simulink model "AFE_3L_DCP_DCN"  (R2013b)
settings: Solver=FixedStepDiscrete  SolverMode=SingleTasking  StartTime=0.0  StopTime=0.9  FixedStep=Tpas  RelTol=1e-3
values from neighbouring files (symbols this model uses):
  ASF3 = .5    (= 0.5)    [AFE_FV_Params.m]    (also in AFE_FV_ParamsPV4.m; Params.m)
  Cbus = 330e-3    (= 0.33)    [AFE_FV_Params.m]    (also in AFE_FV_ParamsPV4.m; Params.m)
  DAFE = 0    [AFE_FV_Params.m]    (also in AFE_FV_ParamsPV4.m; Params.m)
  fmod4Q = 1e3    (= 1000)    [AFE_FV_Params.m]    (also in AFE_FV_ParamsPV4.m; Params.m)
  Freq = 50    [AFE_FV_Params.m]    (also in AFE_FV_ParamsPV4.m; Params.m)
  IAFE3L = (PAFE3L+Numd(2)/Dend(1))/Ts    [AFE_FV_Params.m]    (also in AFE_FV_ParamsPV4.m = (PAFE3L+NumdAFE(2)/DendAFE(1))/Ts; CalcPIAndFilters.m; Params.m = (PAFE3L+NumdAFE(2)/DendAFE(1))/Ts)
  IDCP = (PDCP+Numd(2)/Dend(1))/Tpas    [AFE_FV_Params.m]    (also in AFE_FV_ParamsPV4.m = (PDCP+Numd(2)/Dend(1))/Ts; CalcPIAndFilters.m = (PDCP+Numd(2)/Dend(1))/Ts; Params.m = (PDCP+Numd(2)/Dend(1))/Ts)
  Kac = 1/(Vac*sqrt(2/3))    [AFE_FV_Params.m]    (also in AFE_FV_ParamsPV4.m; Params.m)
  KLPDCP = mat2str(KLPDCP)    [CalcPIAndFilters.m]
  L = .1    (= 0.1)    [AFE_FV_Params.m]    (also in AFE_FV_ParamsPV4.m; Params.m)
  Lac = 8.1487e-04    (= 0.00081487)    [AFE_FV_Params.m]    (also in AFE_FV_ParamsPV4.m; Params.m)
  Lcoup = 1e-6    (= 1e-06)    [AFE_FV_Params.m]    (also in AFE_FV_ParamsPV4.m = 1e-05; Params.m = 1e-05)
  NAFE = 100    [AFE_FV_Params.m]    (also in AFE_FV_ParamsPV4.m; Params.m)
  PAFE3L = Numd(1)/Dend(1)    [AFE_FV_Params.m]    (also in AFE_FV_ParamsPV4.m = NumdAFE(1)/DendAFE(1); CalcPIAndFilters.m; Params.m = NumdAFE(1)/DendAFE(1))
  PDCP = Numd(1)/Dend(1)    [AFE_FV_Params.m]    (also in AFE_FV_ParamsPV4.m; CalcPIAndFilters.m; Params.m)
  R = .28    (= 0.28)    [AFE_FV_Params.m]    (also in AFE_FV_ParamsPV4.m; Params.m)
  Sat3 = 800    [AFE_FV_Params.m]
  TLPDCP = mat2str(TLPDCP)    [CalcPIAndFilters.m]
  Tpas = 1e-6    (= 1e-06)    [AFE_FV_Params.m]    (also in AFE_FV_ParamsPV4.m; Params.m = 1e-05)
  Vac = 2000    [AFE_FV_Params.m]    (also in AFE_FV_ParamsPV4.m; Params.m)
  Vdc = 5000    [AFE_FV_Params.m]    (also in AFE_FV_ParamsPV4.m; Params.m)
undefined symbols (not defined in the file or in its folder): D1, Delta, Rac
libraries: powerlib x80, simulink x36, powerlib_meascontrol x26
(part 2 of 2)

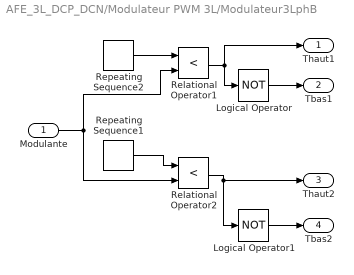
== system AFE_3L_DCP_DCN/Modulateur PWM 3L/Modulateur3LphB ==
  Modulante : Inport
  Logical Operator : Logic  Operator=NOT  AllPortsSameDT=off  OutDataTypeStr=boolean
  Logical Operator1 : Logic  Operator=NOT  AllPortsSameDT=off  OutDataTypeStr=boolean
  Relational Operator1 : RelationalOperator  Operator=<  OutDataTypeStr=boolean
  Relational Operator2 : RelationalOperator  Operator=<  OutDataTypeStr=boolean
  Repeating Sequence1 : simulink/Sources/Repeating Sequence  rep_seq_t=[0 .5/666 1/666]  rep_seq_y=[-1 0 -1]
  Repeating Sequence2 : simulink/Sources/Repeating Sequence  rep_seq_t=[0 .5/666 1/666]  rep_seq_y=[0 1 0]
  Thaut1 : Outport
  Tbas1 : Outport  Port=2
  Thaut2 : Outport  Port=3
  Tbas2 : Outport  Port=4
  wires:
  Repeating Sequence2/1 -> Relational Operator1/1
  Modulante/1 -> Relational Operator1/2, Relational Operator2/2
  Repeating Sequence1/1 -> Relational Operator2/1
  Relational Operator1/1 -> Logical Operator/1, Thaut1/1
  Logical Operator/1 -> Tbas1/1
  Logical Operator1/1 -> Tbas2/1
  Relational Operator2/1 -> Logical Operator1/1, Thaut2/1

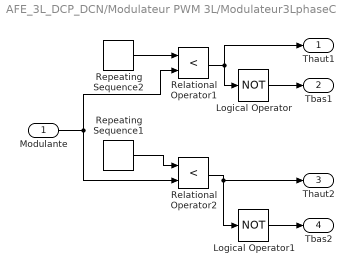
== system AFE_3L_DCP_DCN/Modulateur PWM 3L/Modulateur3LphaseC ==
  Modulante : Inport
  Logical Operator : Logic  Operator=NOT  AllPortsSameDT=off  OutDataTypeStr=boolean
  Logical Operator1 : Logic  Operator=NOT  AllPortsSameDT=off  OutDataTypeStr=boolean
  Relational Operator1 : RelationalOperator  Operator=<  OutDataTypeStr=boolean
  Relational Operator2 : RelationalOperator  Operator=<  OutDataTypeStr=boolean
  Repeating Sequence1 : simulink/Sources/Repeating Sequence  rep_seq_t=[0 .5/666 1/666]  rep_seq_y=[-1 0 -1]
  Repeating Sequence2 : simulink/Sources/Repeating Sequence  rep_seq_t=[0 .5/666 1/666]  rep_seq_y=[0 1 0]
  Thaut1 : Outport
  Tbas1 : Outport  Port=2
  Thaut2 : Outport  Port=3
  Tbas2 : Outport  Port=4
  wires:
  Repeating Sequence2/1 -> Relational Operator1/1
  Modulante/1 -> Relational Operator1/2, Relational Operator2/2
  Repeating Sequence1/1 -> Relational Operator2/1
  Relational Operator1/1 -> Logical Operator/1, Thaut1/1
  Logical Operator/1 -> Tbas1/1
  Logical Operator1/1 -> Tbas2/1
  Relational Operator2/1 -> Logical Operator1/1, Thaut2/1
